simulink model "gm_fpga_block_slrt"  (R2020b)
settings: Solver=FixedStepDiscrete  StartTime=0.0  StopTime=5  FixedStep=5e-5  RelTol=1e-3
PostLoadFcn:
  | try
  | cell = struct2cell(dir(fullfile(speedgoatroot_hdlb, 'hdlsrc', 'quadrature', '*.vhd')));
  | addSourceFiles = strjoin(fullfile(cell(2,:),cell(1,:)), ';');
  | hdlset_param('quadrature_example_hdlc/DUT Quadrature', 'IPCoreAdditionalFiles', addSourceFiles);
  | end
undefined symbols (not defined in the file): FPGA, fpga_block, IO334
libraries: speedgoatlib_hdlCoder_IO3xx x11, eePwmGenerator x3, slrealtimeutilitieslib x1, pwm_cpulib x1, quadrature_cpulib x1
settings Model: ModifiedByFormat=Speedgoat GmbH  Creator=Speedgoat GmbH  LastModifiedBy=Speedgoat GmbH
settings SolverCC: ConcurrentTasks=on  PositivePriorityOrder=on
settings DataIOCC: ReturnWorkspaceOutputs=off
settings OptimizationCC: BlockReduction=off  ConditionallyExecuteInputs=off  DefaultParameterBehavior=Inlined  OptimizeBlockIOStorage=off
settings DebuggingCC: AlgebraicLoopMsg=error  InheritedTsInSrcMsg=none  SingleTaskRateTransMsg=error  TasksWithSamePriorityMsg=none  ParameterOverflowMsg=warning  ParameterPrecisionLossMsg=none  PregeneratedLibrarySubsystemCodeDiagnostic=none  ArithmeticOperatorsInVariantConditions=warning
settings HardwareCC: ProdBitPerLong=64  ProdLongLongMode=on  ProdHWDeviceType=Intel->x86-64 (Linux 64)  TargetBitPerPointer=64  TargetBitPerSizeT=64  TargetBitPerPtrDiffT=64  TargetLongLongMode=on  TargetIntDivRoundTo=Zero  TargetEndianess=LittleEndian  TargetWordSize=64  TargetHWDeviceType=Custom Processor->MATLAB Host Computer
settings SFSimCC: SimUseLocalCustomCode=off  CustomCodeUndefinedFunction=UseInterfaceOnly
settings RTWCC: Description=Simulink Real-Time  SystemTargetFile=slrealtime.tlc  TemplateMakefile=slrealtime_default_tmf  RTWUseLocalCustomCode=off  Toolchain=Simulink Real-Time Toolchain  BuildConfiguration=Faster Runs  CodeExecutionProfiling=on  TargetLang=C++

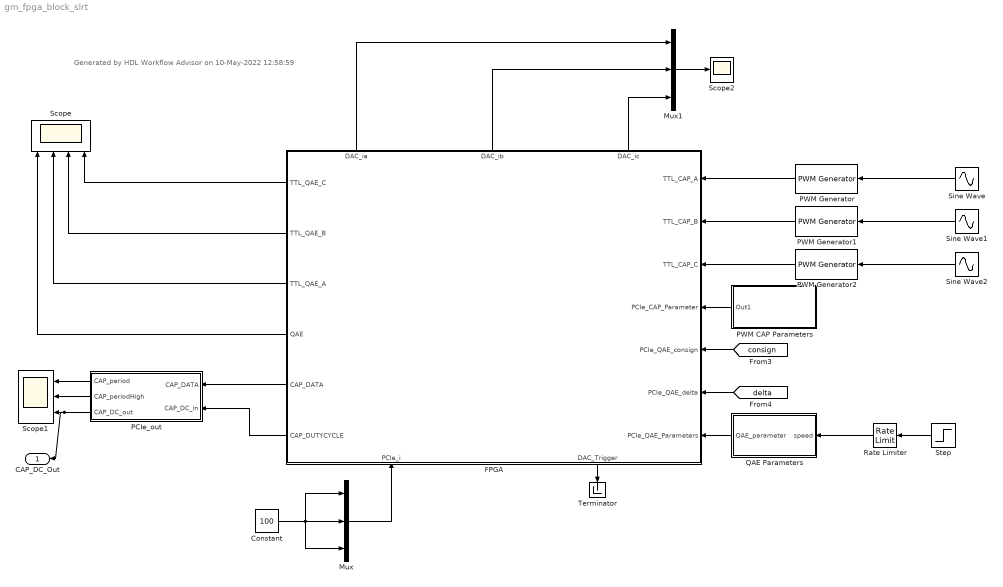
== system gm_fpga_block_slrt ==
  note: Generated by HDL Workflow Advisor on 10-May-2022 12:58:59
  Constant : Constant  Value=100  OutDataTypeStr=int16  SampleTime=5e-5
  FPGA : Subsystem  mask(Speedgoat IO334-325k Interface Block){module_id=1, slot=-1, ts=-1, OutputRange=Auto (same as ADC), PullRPort0=pull-up 3.3V, VioPort0=3.3V, PullRPort1=pull-up 3.3V, VioPort1=3.3V, PullRPort2=pull-up 3.3V, VioPort2=3.3V, PullRPort3=pull-up 3.3V, VioPort3=3.3V, PullRPort4=pull-up 3.3V, VioPort4=3.3V, PullRPort5=pull-up 3.3V, VioPort5=3.3V, PullRPort6=pull-up 3.3V, VioPort6=3.3V, FpgaFreq=100}
      mask prompts: module_id "FPGA Module Identifier:"; slot "PCI slot (-1: autosearch):"; ts "Sample time:"; OutputRange "DAC Voltage Range:"; PullRPort0 "pull resistor"; VioPort0 "I/O voltage"; PullRPort1 "pull resistor"; VioPort1 "I/O voltage"; PullRPort2 "pull resistor"; VioPort2 "I/O voltage"; PullRPort3 "pull resistor"; VioPort3 "I/O voltage"; PullRPort4 "pull resistor"; VioPort4 "I/O voltage"; PullRPort5 "pull resistor"; VioPort5 "I/O voltage"; PullRPort6 "pull resistor"; VioPort6 "I/O voltage"; FpgaFreq "FPGA Frequency [MHz]"
      mask help: Simulink Real-Time Interface Block for Speedgoat IO334-325k.
      mask init:
      | hdlslrt.backend.mfpgaparameters;
      settings: PortSchema="{\"entries\":[{\"content\":{\"sides\":[{\"content\":{\"connectorIds\":[\"In1\",\"In2\",\"In3\",\"In4\",\"In5\",\"In6\",\"In7\"]},\"type\":\"ConnectorPlacement.EquallySpacedRectSide\",\"uuid\":\"e6984190-0c70-4c87-a85a-93b5ecf8c70e\"},{\"content\":{\"connectorIds\":[\"Out1\",\"Out2\",\"Out3\",\"Out4\",\"Out5\",\"Out6\"],\"side\":\"RIGHT\"},\"type\":\"ConnectorPlacement.EquallySpacedRectSide\",\"uuid\":\"15751016-c591-4c93-a1ea-9b92ed7cff5f\"},{\"content\":{\"connectorIds\":[\"Out8\",\"Out9\",\"Out10\"],\"side\":\"TOP\"},\"type\":\"ConnectorPlacement.EquallySpacedRectSide\",\"uuid\":\"0ed2d626-9fdd-4a40-8e61-e2e65c1699d5\"},{\"content\":{\"connectorIds\":[\"Out7\",\"In8\"],\"side\":\"BOTTOM\"},\"type\":\"ConnectorPlacement.EquallySpacedRectSide\",\"uuid\":\"ca9e0c29-7634-4998-8fab-ad91c1afd2ab\"},{\"content\":{\"connectorIds\":[],\"side\":\"HIDDEN\"},\"type\":\"ConnectorPlacement.EquallySpacedRectSide\",\"uuid\":\"82c879c3-3b90-47c5-9b46-55d1ced3d9d8\"}]},\"type\":\"ConnectorPlacement.EquallySpacedConnector\",\"uuid\":\"f7068230-82ff-4dc7-8776-ae1c0daadd88\"}],\"packageUris\":[\"http://schema.mathworks.com/mf0/Connector/R2020b\"],\"version\":\"1.0\"}"
      mask Help: eval('speedgoatdoc_hdlc')
      mask TypeOptions OutputRange: IO334 DAC Setup/OutputRange
      mask TypeOptions PullRPort0: Port Settings -2x/PullRPort0
      mask Callback PullRPort0: sg_fpga_HDLCoder_io3xx_2x_m(2)
      mask TypeOptions VioPort0: Port Settings -2x/VioPort0
      mask Callback VioPort0: sg_fpga_HDLCoder_io3xx_2x_m(2)
      mask TypeOptions PullRPort1: Port Settings -2x/PullRPort1
      mask Callback PullRPort1: sg_fpga_HDLCoder_io3xx_2x_m(2)
      mask TypeOptions VioPort1: Port Settings -2x/VioPort1
      mask Callback VioPort1: sg_fpga_HDLCoder_io3xx_2x_m(2)
      mask TypeOptions PullRPort2: Port Settings -2x/PullRPort2
      mask Callback PullRPort2: sg_fpga_HDLCoder_io3xx_2x_m(2)
      mask TypeOptions VioPort2: Port Settings -2x/VioPort2
      mask Callback VioPort2: sg_fpga_HDLCoder_io3xx_2x_m(2)
      mask TypeOptions PullRPort3: Port Settings -2x/PullRPort3
      mask Callback PullRPort3: sg_fpga_HDLCoder_io3xx_2x_m(2)
      mask TypeOptions VioPort3: Port Settings -2x/VioPort3
      mask Callback VioPort3: sg_fpga_HDLCoder_io3xx_2x_m(2)
      mask TypeOptions PullRPort4: Port Settings -2x/PullRPort4
      mask Callback PullRPort4: sg_fpga_HDLCoder_io3xx_2x_m(2)
      mask TypeOptions VioPort4: Port Settings -2x/VioPort4
      mask Callback VioPort4: sg_fpga_HDLCoder_io3xx_2x_m(2)
      mask TypeOptions PullRPort5: Port Settings -2x/PullRPort5
      mask Callback PullRPort5: sg_fpga_HDLCoder_io3xx_2x_m(2)
      mask TypeOptions VioPort5: Port Settings -2x/VioPort5
      mask Callback VioPort5: sg_fpga_HDLCoder_io3xx_2x_m(2)
      mask TypeOptions PullRPort6: Port Settings -2x/PullRPort6
      mask Callback PullRPort6: sg_fpga_HDLCoder_io3xx_2x_m(2)
      mask TypeOptions VioPort6: Port Settings -2x/VioPort6
      mask Callback VioPort6: sg_fpga_HDLCoder_io3xx_2x_m(2)
      mask DialogControl AnalogOutput Prompt: Analog Output
      mask DialogControl IO33421 Prompt: IO334-21
      mask DialogControl port1 Prompt: Port 1
      mask DialogControl port2 Prompt: Port 2
      mask DialogControl port3 Prompt: Port 3
      mask DialogControl port4 Prompt: Port 4
      mask DialogControl port5 Prompt: Port 5
      mask DialogControl port6 Prompt: Port 6
      mask DialogControl port7 Prompt: Port 7
      mask Display:
      | SetupBlkPath = find_system(gcb, 'LookUnderMasks', 'all', 'FollowLinks', 'on', 'regexp', 'on', 'Name', 'IO3(\d|x){2}\s+Setup' );
      | SetupBlkPath = SetupBlkPath{1};
      | TS = get_param(SetupBlkPath,'timestamp_mcs');
      | disp(sprintf('Speedgoat IO334-325k\nFPGA I/O Module\n\nTimestamp\n%s\n\nReference Design\nVersion 2.1\n\nMatlab R2020b\n\nPCIe Link Width: X4\nRear Plugin: -21\nAurora Mode: None\nAurora Byteswap: true\n', TS))
  Mux : Mux  Inputs=3
  Mux1 : Mux  Inputs=3
  PCIe_out : Subsystem
  PWM CAP Parameters : Subsystem
  PWM Generator : eePwmGenerator/PWM Generator  CarrCount=Up  Tper=0.01  Ts=2e-4
  PWM Generator1 : eePwmGenerator/PWM Generator  CarrCount=Up  Tper=0.01  Ts=2e-4
  PWM Generator2 : eePwmGenerator/PWM Generator  CarrCount=Up  Tper=0.01  Ts=2e-4
  QAE Parameters : Subsystem
  Rate Limiter : RateLimiter  RisingSlewLimit=50  FallingSlewLimit=-50  SampleTimeMode=inherited
  Scope : Scope  NumInputPorts=4
  Scope1 : Scope  NumInputPorts=3
  Scope2 : Scope
  Sine Wave : Sin  Amplitude=0.5  Bias=0.5  Frequency=2*pi
  Sine Wave1 : Sin  Amplitude=0.5  Bias=0.5  Frequency=2*pi  Phase=2*pi/3
  Sine Wave2 : Sin  Amplitude=0.5  Bias=0.5  Frequency=2*pi  Phase=4*pi/3
  Step : Step  Time=0.1  After=100
  Terminator : Terminator
  CAP_DC_Out : Outport  VectorParamsAs1DForOutWhenUnconnected=off
  wires:
  Mux/1 -> FPGA/8(PCIe_i)
  FPGA/7(DAC_Trigger) -> Terminator/1
  FPGA/10(DAC_ia) -> Mux1/1
  FPGA/9(DAC_ib) -> Mux1/2
  FPGA/8(DAC_ic) -> Mux1/3
  Mux1/1 -> Scope2/1
  Constant/1 -> Mux/1, Mux/2, Mux/3
  Sine Wave2/1 -> PWM Generator2/1
  Sine Wave1/1 -> PWM Generator1/1
  Sine Wave/1 -> PWM Generator/1
  Step/1 -> Rate Limiter/1
  Rate Limiter/1 -> QAE Parameters/1(speed)
  FPGA/6(CAP_DUTYCYCLE) -> PCIe_out/2(CAP_DC_in)
  FPGA/5(CAP_DATA) -> PCIe_out/1(CAP_DATA)
  FPGA/1(TTL_QAE_C) -> Scope/4
  FPGA/2(TTL_QAE_B) -> Scope/3
  FPGA/3(TTL_QAE_A) -> Scope/2
  FPGA/4(QAE) -> Scope/1
  PWM CAP Parameters/1(Out1) -> FPGA/4(PCIe_CAP_Parameter)
  PWM Generator2/1 -> FPGA/3(TTL_CAP_C)
  PWM Generator1/1 -> FPGA/2(TTL_CAP_B)
  PWM Generator/1 -> FPGA/1(TTL_CAP_A)
  [delta] -> FPGA/6(PCIe_QAE_delta)
  [consign] -> FPGA/5(PCIe_QAE_consign)
  QAE Parameters/1(QAE_parameter) -> FPGA/7(PCIe_QAE_Parameters)
  PCIe_out/3(CAP_DC_out) -> CAP_DC_Out/1, Scope1/3
  PCIe_out/2(CAP_periodHigh) -> Scope1/2
  PCIe_out/1(CAP_period) -> Scope1/1

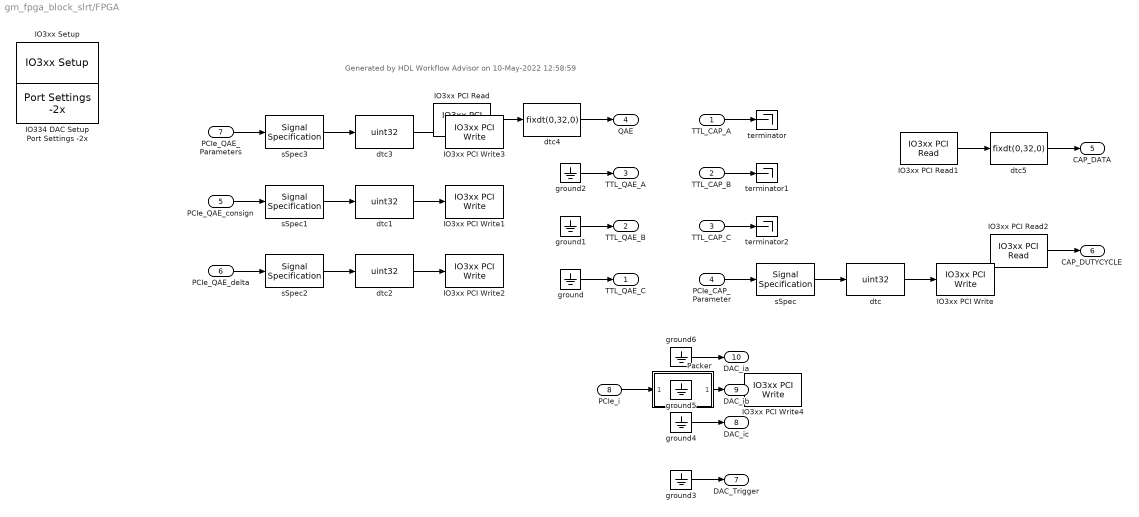
== system gm_fpga_block_slrt/FPGA ==
  note: Generated by HDL Workflow Advisor on 10-May-2022 12:58:59
  TTL_CAP_A : Inport
  TTL_CAP_B : Inport  Port=2
  TTL_CAP_C : Inport  Port=3
  PCIe_CAP_Parameter : Inport  Port=4
  PCIe_QAE_consign : Inport  Port=5
  PCIe_QAE_delta : Inport  Port=6
  PCIe_QAE_Parameters : Inport  Port=7
  PCIe_i : Inport  Port=8
  IO334 DAC Setup : speedgoatlib_hdlCoder_IO3xx/IO334 DAC Setup  module_id=module_id  OutputRange=Auto (same as ADC)
  IO3xx PCI Read : speedgoatlib_hdlCoder_IO3xx/IO3xx PCI Read  device_id=deviceIdx  module_id=module_id  board_type=IO3xx  port_name=QAE  port_offset=hex2dec('138')  port_type=uint32  port_dim=1  strobe=0  sample_time=ts
  IO3xx PCI Read1 : speedgoatlib_hdlCoder_IO3xx/IO3xx PCI Read  device_id=deviceIdx  module_id=module_id  board_type=IO3xx  port_name=CAP_DATA  port_offset=hex2dec('200')  port_type=uint32  port_dim=18  strobe=hex2dec('280')  sample_time=ts
  IO3xx PCI Read2 : speedgoatlib_hdlCoder_IO3xx/IO3xx PCI Read  device_id=deviceIdx  module_id=module_id  board_type=IO3xx  port_name=CAP_DUTYCYCLE  port_offset=hex2dec('170')  port_type=single  port_dim=3  strobe=hex2dec('180')  sample_time=ts
  IO3xx PCI Write : speedgoatlib_hdlCoder_IO3xx/IO3xx PCI Write  device_id=deviceIdx  module_id=module_id  board_type=IO3xx  port_name=PCIe_CAP_Parameter  port_offset=hex2dec('140')  port_type=uint32  port_dim=3  strobe=hex2dec('150')  sample_time=ts
  IO3xx PCI Write1 : speedgoatlib_hdlCoder_IO3xx/IO3xx PCI Write  device_id=deviceIdx  module_id=module_id  board_type=IO3xx  port_name=PCIe_QAE_consign  port_offset=hex2dec('124')  port_type=uint32  port_dim=1  strobe=0  sample_time=ts
  IO3xx PCI Write2 : speedgoatlib_hdlCoder_IO3xx/IO3xx PCI Write  device_id=deviceIdx  module_id=module_id  board_type=IO3xx  port_name=PCIe_QAE_delta  port_offset=hex2dec('128')  port_type=uint32  port_dim=1  strobe=0  sample_time=ts
  IO3xx PCI Write3 : speedgoatlib_hdlCoder_IO3xx/IO3xx PCI Write  device_id=deviceIdx  module_id=module_id  board_type=IO3xx  port_name=PCIe_QAE_Parameters  port_offset=hex2dec('100')  port_type=uint32  port_dim=7  strobe=hex2dec('120')  sample_time=ts
  IO3xx PCI Write4 : speedgoatlib_hdlCoder_IO3xx/IO3xx PCI Write  device_id=deviceIdx  module_id=module_id  board_type=IO3xx  port_name=PCIe_i  port_offset=hex2dec('158')  port_type=uint32  port_dim=2  strobe=hex2dec('160')  sample_time=ts
  IO3xx Setup : speedgoatlib_hdlCoder_IO3xx/IO3xx Setup  mdl_ss_name=fpga_block/FPGA  board_type=IO334-325k  fpga_sync_mode=on  reset_mode=on  device_id=deviceIdx  module_id=module_id  pci_slot=slot  fpga_mat_file=hdl_prj\hdlsrc\fpga_block\FPGA.mat  timestamp_mcs=05/09/22 19:31:06  timestamp=2205091845  tsreg=hex2dec('8')  bsf_file=FPGA_2205091845.mcs  mcs=0
  Packer : Subsystem
  Port Settings -2x : speedgoatlib_hdlCoder_IO3xx/Port Settings -2x  module_id=module_id  rearIO=-21  PullRPort0=pull-up 3.3V  VioPort0=3.3V  PullRPort1=pull-up 3.3V  VioPort1=3.3V  PullRPort2=pull-up 3.3V  VioPort2=3.3V  PullRPort3=pull-up 3.3V  VioPort3=3.3V  PullRPort4=pull-up 3.3V  VioPort4=3.3V  PullRPort5=pull-up 3.3V  VioPort5=3.3V  PullRPort6=pull-up 3.3V  VioPort6=3.3V
  dtc{,1..3} (4 alike) : DataTypeConversion  OutDataTypeStr=uint32  ConvertRealWorld=Stored Integer (SI)  RndMeth=Zero
  dtc4 : DataTypeConversion  OutDataTypeStr=fixdt(0,32,0)  ConvertRealWorld=Stored Integer (SI)  RndMeth=Zero
  dtc5 : DataTypeConversion  OutDataTypeStr=fixdt(0,32,0)  ConvertRealWorld=Stored Integer (SI)  RndMeth=Zero
  ground{,1..6} (7 alike) : Ground
  sSpec : SignalSpecification  OutDataTypeStr=fixdt(0,32,0)
  sSpec1 : SignalSpecification  OutDataTypeStr=fixdt(0,32,0)
  sSpec2 : SignalSpecification  OutDataTypeStr=fixdt(1,32,0)
  sSpec3 : SignalSpecification  OutDataTypeStr=fixdt(0,32,0)
  terminator : Terminator
  terminator1 : Terminator
  terminator2 : Terminator
  TTL_QAE_C : Outport
  TTL_QAE_B : Outport  Port=2
  TTL_QAE_A : Outport  Port=3
  QAE : Outport  Port=4
  CAP_DATA : Outport  Port=5
  CAP_DUTYCYCLE : Outport  Port=6
  DAC_Trigger : Outport  Port=7
  DAC_ic : Outport  Port=8
  DAC_ib : Outport  Port=9
  DAC_ia : Outport  Port=10
  wires:
  TTL_CAP_A/1 -> terminator/1
  TTL_CAP_B/1 -> terminator1/1
  TTL_CAP_C/1 -> terminator2/1
  PCIe_CAP_Parameter/1 -> sSpec/1
  sSpec/1 -> dtc/1
  dtc/1 -> IO3xx PCI Write/1
  PCIe_QAE_consign/1 -> sSpec1/1
  sSpec1/1 -> dtc1/1
  dtc1/1 -> IO3xx PCI Write1/1
  PCIe_QAE_delta/1 -> sSpec2/1
  sSpec2/1 -> dtc2/1
  dtc2/1 -> IO3xx PCI Write2/1
  PCIe_QAE_Parameters/1 -> sSpec3/1
  sSpec3/1 -> dtc3/1
  dtc3/1 -> IO3xx PCI Write3/1
  PCIe_i/1 -> Packer/1(unpacked)
  Packer/1(packed) -> IO3xx PCI Write4/1
  ground/1 -> TTL_QAE_C/1
  ground1/1 -> TTL_QAE_B/1
  ground2/1 -> TTL_QAE_A/1
  dtc4/1 -> QAE/1
  IO3xx PCI Read/1 -> dtc4/1
  dtc5/1 -> CAP_DATA/1
  IO3xx PCI Read1/1 -> dtc5/1
  IO3xx PCI Read2/1 -> CAP_DUTYCYCLE/1
  ground3/1 -> DAC_Trigger/1
  ground4/1 -> DAC_ic/1
  ground5/1 -> DAC_ib/1
  ground6/1 -> DAC_ia/1

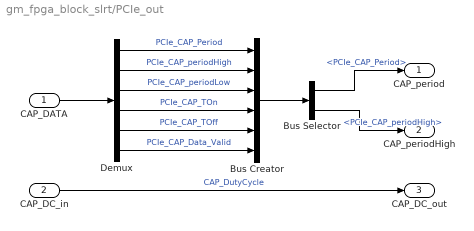
== system gm_fpga_block_slrt/PCIe_out ==
  CAP_DATA : Inport
  CAP_DC_in : Inport  Port=2
  Bus Creator : BusCreator  Inputs=6
  Bus Selector : BusSelector  OutputSignals=PCIe_CAP_Period,PCIe_CAP_periodHigh
  Demux : Demux  Outputs=6
  CAP_period : Outport
  CAP_periodHigh : Outport  Port=2
  CAP_DC_out : Outport  Port=3
  wires:
  CAP_DATA/1 -> Demux/1
  Demux/5 -> Bus Creator/5  "PCIe_CAP_TOff"
  Demux/1 -> Bus Creator/1  "PCIe_CAP_Period"
  Bus Creator/1 -> Bus Selector/1
  Demux/4 -> Bus Creator/4  "PCIe_CAP_TOn"
  Demux/2 -> Bus Creator/2  "PCIe_CAP_periodHigh"
  Demux/3 -> Bus Creator/3  "PCIe_CAP_periodLow"
  Demux/6 -> Bus Creator/6  "PCIe_CAP_Data_Valid"
  Bus Selector/1 -> CAP_period/1  "<PCIe_CAP_Period>"
  Bus Selector/2 -> CAP_periodHigh/1  "<PCIe_CAP_periodHigh>"
  CAP_DC_in/1 -> CAP_DC_out/1  "CAP_DutyCycle"

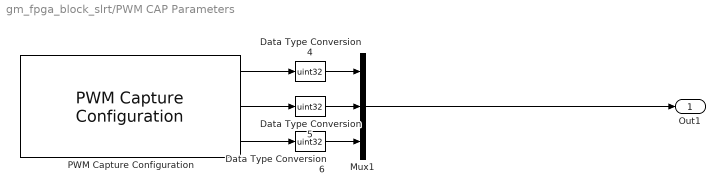
== system gm_fpga_block_slrt/PWM CAP Parameters ==
  Data Type Conversion4 : DataTypeConversion  OutDataTypeStr=uint32
  Data Type Conversion5 : DataTypeConversion  OutDataTypeStr=uint32
  Data Type Conversion6 : DataTypeConversion  OutDataTypeStr=uint32
  Mux1 : Mux  Inputs=3
  PWM Capture Configuration : pwm_cpulib/PWM Capture Configuration  FPGA_freq=100e6  n_channels=1  captureMode=High transitions triggered  captureTimeout=0  PWM_pattern_en=off
      settings: SourceProductName=Simulink Real-Time: Speedgoat HDL Blockset
  Out1 : Outport
  wires:
  Data Type Conversion5/1 -> Mux1/2
  PWM Capture Configuration/3 -> Data Type Conversion6/1
  Data Type Conversion4/1 -> Mux1/1
  PWM Capture Configuration/1 -> Data Type Conversion4/1
  Mux1/1 -> Out1/1
  Data Type Conversion6/1 -> Mux1/3
  PWM Capture Configuration/2 -> Data Type Conversion5/1

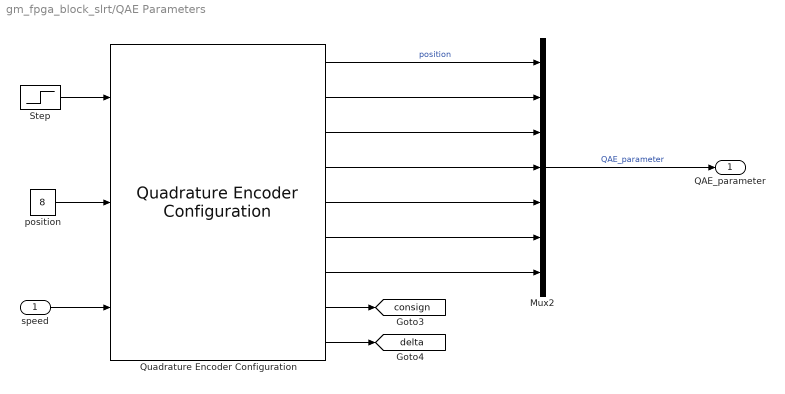
== system gm_fpga_block_slrt/QAE Parameters ==
  speed : Inport
  Mux2 : Mux  Inputs=7
  Quadrature Encoder Configuration : quadrature_cpulib/Quadrature Encoder Configuration  fpgaFreq=100e6  n_channels=1  numSeg=[16]  phaseAngle=90  initPos=[0]  freeWheel=on
      settings: SourceProductName=Simulink Real-Time: Speedgoat HDL Blockset
  Step : Step  Time=0.002
  position : Constant  Value=8  SampleTime=-1
  QAE_parameter : Outport
  tag scope: consign=global, delta=global
  wires:
  Mux2/1 -> QAE_parameter/1  "QAE_parameter"
  Quadrature Encoder Configuration/4 -> Mux2/4
  Quadrature Encoder Configuration/7 -> Mux2/7
  Step/1 -> Quadrature Encoder Configuration/1
  Quadrature Encoder Configuration/1 -> Mux2/1  "position"
  speed/1 -> Quadrature Encoder Configuration/3
  Quadrature Encoder Configuration/9 -> [delta]
  Quadrature Encoder Configuration/3 -> Mux2/3
  Quadrature Encoder Configuration/8 -> [consign]
  position/1 -> Quadrature Encoder Configuration/2
  Quadrature Encoder Configuration/6 -> Mux2/6
  Quadrature Encoder Configuration/5 -> Mux2/5
  Quadrature Encoder Configuration/2 -> Mux2/2

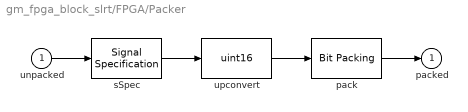
== system gm_fpga_block_slrt/FPGA/Packer ==
  unpacked : Inport
  pack : slrealtimeutilitieslib/Bit Packing  MaskBitPatterns={[0:15 16:31 32:47 ]}  MaskPackDataType=uint32  MaskPackDataSize=2
      settings: SourceProductBaseCode=XP
  sSpec : SignalSpecification  OutDataTypeStr=fixdt(1,16,0)
  upconvert : DataTypeConversion  OutDataTypeStr=uint16  ConvertRealWorld=Stored Integer (SI)  RndMeth=Zero
  packed : Outport
  wires:
  unpacked/1 -> sSpec/1
  sSpec/1 -> upconvert/1
  upconvert/1 -> pack/1
  pack/1 -> packed/1
